simulink model "MSFartoystyring_path"  (R2018a)
settings: Solver=ode45  StartTime=tstart  StopTime=tstop  RelTol=1e-3  EnableMultiTasking=on
values from neighbouring files (symbols this model uses):
  c = 0    [run_heading.m]    (also in run_heading_controller.m = 1; run_heading_model.m; run_path.m = 1; run_path_crab.m)
  K_d = 2*zeta*w_n*(m + K_m) - d    [run_heading_controller.m]    (also in run_path.m)
  K_i = w_n / 10 * K_p    [run_heading_controller.m]    (also in run_path.m)
  K_p = (m+K_m)*w_n^2 - k    [run_heading_controller.m]    (also in run_path.m)
  n_max = (85*2*pi)/60    (= 8.90117918517)    [run_heading.m]    (also in run_heading_controller.m; run_heading_model.m; run_path.m; run_path_crab.m)
  p0 = zeros(2,1)    [run_heading.m]    (also in run_heading_controller.m; run_heading_model.m; run_path.m = [1000; 700]; run_path_crab.m = [1000; 700])
  psi0 = 0    [run_heading.m]    (also in run_heading_controller.m; run_heading_model.m; run_path.m = deg2rad(60); run_path_crab.m = deg2rad(-135))
  psi_d = deg2rad(10)    [run_path.m]    (also in run_path_crab.m; run_track.m)
  r0 = 0    [run_heading.m]    (also in run_heading_controller.m; run_heading_model.m; run_path.m; run_path_crab.m)
  tsamp = 10    [run_heading.m]    (also in run_heading_controller.m = 1; run_heading_model.m = 1; run_path.m; run_path_crab.m)
  v0 = [6.63 0]'    [run_heading.m]    (also in run_heading_controller.m; run_heading_model.m; run_path.m; run_path_crab.m)
undefined symbols (not defined in the file or in its folder): msfartoystyring, WP
libraries: simulink x2
settings Model: ExtModeAutoUpdateStatusClock=off  Creator=christh  LastModifiedBy=nicho
settings DataIOCC: LimitDataPoints=on  SaveFormat=Array  SignalLoggingSaveFormat=ModelDataLogs
settings OptimizationCC: ExpressionDepthLimit=2147483647  InitFltsAndDblsToZero=on  LifeSpan=inf
settings DebuggingCC: UnderspecifiedInitializationDetection=Classic  MergeDetectMultiDrivingBlocksExec=none  SolverPrmCheckMsg=warning  FcnCallInpInsideContextMsg=warning  StateNameClashWarn=warning  SFUnexpectedBacktrackingDiag=warning  SFNoUnconditionalDefaultTransitionDiag=warning  SFExecutionAtInitializationDiag=none
settings HardwareCC: ProdBitPerPointer=32  ProdBitPerSizeT=32  ProdBitPerPtrDiffT=32  ProdLargestAtomicFloat=None  ProdIntDivRoundTo=Undefined  ProdEndianess=Unspecified  ProdWordSize=32  ProdHWDeviceType=32-bit Generic
settings ModelReferenceCC: PropagateSignalLabelsOutOfModel=off
settings CodeAppCC: StateflowObjectComments=on
settings GRTTargetCC: TargetLangStandard=C89/C90 (ANSI)  GeneratePreprocessorConditionals=Disable all  CombineOutputUpdateFcns=off  GRTInterface=on
settings ConfigComp: CovMetricSettings=dw  CovHtmlReporting=on  CovSaveCumulativeToWorkspaceVar=on  CovSaveSingleToWorkspaceVar=on  CovExternalEMLEnable=off

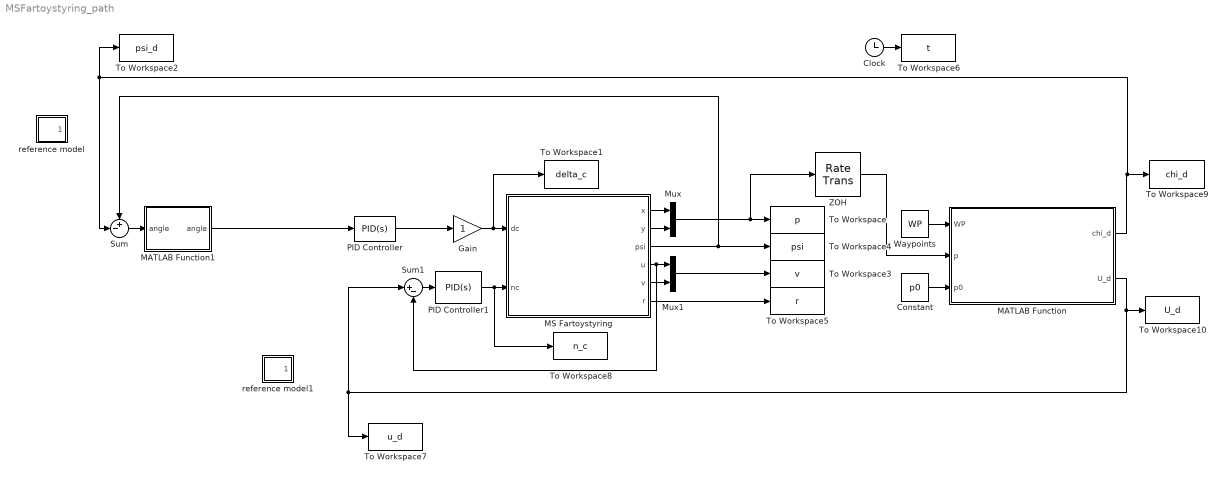
== system MSFartoystyring_path ==
  Clock : Clock
  Constant : Constant  Value=p0
  Gain : Gain
  MATLAB Function : MATLAB Function  TreatAsAtomicUnit=on
  MATLAB Function1 : MATLAB Function  TreatAsAtomicUnit=on
  MS Fartoystyring : Subsystem  mask(MS Fartoystyring for Assignment 3 G&C){x0=p0(1), y0=p0(2), u0=v0(1), v0=v0(2), psi0=psi0, r0=r0, c=c}
      mask prompts: x0 "x(t0) (m)"; y0 "y(t0) (m)"; u0 "u(t0) (m/s)"; v0 "v(t0) (m/s)"; psi0 "psi(t0) (rad)"; r0 "r(t0) (rad/s)"; c "current (0 or 1)"
      mask help:
      | Block corresponding to Figure 1 in the assignment text. Gives the response of the ship.
      |
      | The design speed of MS Fartoystyring is u=8.23 m/s.
      |
      | Input:
      | dc: commanded rudder (rad), dmax=25*pi/180
      | nc: commanded shaft speed (rad/s), nmax=85*2*pi/60
      |
      | Output:
      | x: north pos (m)
      | y: east pos (m)
      | u: surge (m/s)
      | v: sway (m/s)
      | psi: heading (rad)
      | r: yaw (rad/s)
      mask Help: Comments, bugs and help requests can be directed to the TA. Email on course website.
  Mux : Mux  Inputs=2
  Mux1 : Mux  Inputs=2
  PID Controller : simulink/Continuous/PID Controller  Controller=PID  TimeDomain=Continuous-time  SampleTime=-1  IntegratorMethod=Forward Euler  FilterMethod=Forward Euler  Form=Parallel  UseFilter=on  ControllerParametersSource=internal  P=K_p  I=K_i  D=K_d  N=0.0237516416222345  InitialConditionSource=internal  InitialConditionForIntegrator=0  InitialConditionForFilter=0  ExternalReset=none  LimitOutput=on  UpperSaturationLimit=inf  LowerSaturationLimit=-inf  LinearizeAsGain=on  AntiWindupMode=clamping  Kb=1  TrackingMode=off  Kt=1  PParamMin=[]  PParamMax=[]  IParamMin=[]  IParamMax=[]  DParamMin=[]  DParamMax=[]  NParamMin=[]  NParamMax=[]  KbParamMin=[]  KbParamMax=[]  KtParamMin=[]  KtParamMax=[]  POutMin=[]  POutMax=[]  IOutMin=[]  IOutMax=[]  DOutMin=[]  DOutMax=[]  NOutMin=[]  NOutMax=[]  KbOutMin=[]  KbOutMax=[]  KtOutMin=[]  KtOutMax=[]  IntegratorOutMin=[]  IntegratorOutMax=[]  FilterOutMin=[]  FilterOutMax=[]  SumOutMin=[]  SumOutMax=[]  SumI1OutMin=[]  SumI1OutMax=[]  SumI2OutMin=[]  SumI2OutMax=[]  SumI3OutMin=[]  SumI3OutMax=[]  SumDOutMin=[]  SumDOutMax=[]  SaturationOutMin=[]  SaturationOutMax=[]  IntegratorContinuousStateAttributes=''  IntegratorStateMustResolveToSignalObject=off  IntegratorRTWStateStorageClass=Auto  FilterContinuousStateAttributes=''  FilterStateMustResolveToSignalObject=off  FilterRTWStateStorageClass=Auto  DifferentiatorICPrevScaledInput=0  DifferentiatorOutMin=[]  DifferentiatorOutMax=[]  FilterDiffOutCoefMin=[]  FilterDiffOutCoefMax=[]  SumDenOutMin=[]  SumDenOutMax=[]  SumNumOutMin=[]  SumNumOutMax=[]  ReciprocalOutMin=[]  ReciprocalOutMax=[]  DivideOutMin=[]  DivideOutMax=[]  TunerSelectOption=Transfer Function Based (PID Tuner App)
  PID Controller1 : simulink/Continuous/PID Controller  Controller=PID  TimeDomain=Continuous-time  SampleTime=-1  IntegratorMethod=Forward Euler  FilterMethod=Forward Euler  Form=Parallel  UseFilter=on  ControllerParametersSource=internal  P=10  I=2  D=0  N=0.00193532941073824  InitialConditionSource=internal  InitialConditionForIntegrator=0  InitialConditionForFilter=0  ExternalReset=none  LimitOutput=on  UpperSaturationLimit=n_max  LowerSaturationLimit=-n_max  LinearizeAsGain=on  AntiWindupMode=clamping  Kb=1  TrackingMode=off  Kt=1  PParamMin=[]  PParamMax=[]  IParamMin=[]  IParamMax=[]  DParamMin=[]  DParamMax=[]  NParamMin=[]  NParamMax=[]  KbParamMin=[]  KbParamMax=[]  KtParamMin=[]  KtParamMax=[]  POutMin=[]  POutMax=[]  IOutMin=[]  IOutMax=[]  DOutMin=[]  DOutMax=[]  NOutMin=[]  NOutMax=[]  KbOutMin=[]  KbOutMax=[]  KtOutMin=[]  KtOutMax=[]  IntegratorOutMin=[]  IntegratorOutMax=[]  FilterOutMin=[]  FilterOutMax=[]  SumOutMin=[]  SumOutMax=[]  SumI1OutMin=[]  SumI1OutMax=[]  SumI2OutMin=[]  SumI2OutMax=[]  SumI3OutMin=[]  SumI3OutMax=[]  SumDOutMin=[]  SumDOutMax=[]  SaturationOutMin=[]  SaturationOutMax=[]  IntegratorContinuousStateAttributes=''  IntegratorStateMustResolveToSignalObject=off  IntegratorRTWStateStorageClass=Auto  FilterContinuousStateAttributes=''  FilterStateMustResolveToSignalObject=off  FilterRTWStateStorageClass=Auto  DifferentiatorICPrevScaledInput=0  DifferentiatorOutMin=[]  DifferentiatorOutMax=[]  FilterDiffOutCoefMin=[]  FilterDiffOutCoefMax=[]  SumDenOutMin=[]  SumDenOutMax=[]  SumNumOutMin=[]  SumNumOutMax=[]  ReciprocalOutMin=[]  ReciprocalOutMax=[]  DivideOutMin=[]  DivideOutMax=[]  TunerSelectOption=Transfer Function Based (PID Tuner App)
  Sum : Sum  Inputs=+-|
  Sum1 : Sum  Inputs=|+-
  To Workspace : ToWorkspace  VariableName=p  SampleTime=tsamp
  To Workspace1 : ToWorkspace  VariableName=delta_c  SampleTime=tsamp
  To Workspace10 : ToWorkspace  VariableName=U_d  SaveFormat=Timeseries  SampleTime=-1
  To Workspace2 : ToWorkspace  VariableName=psi_d  SampleTime=tsamp
  To Workspace3 : ToWorkspace  VariableName=v  SampleTime=tsamp
  To Workspace4 : ToWorkspace  VariableName=psi  SampleTime=tsamp
  To Workspace5 : ToWorkspace  VariableName=r  SampleTime=tsamp
  To Workspace6 : ToWorkspace  VariableName=t  SampleTime=tsamp
  To Workspace7 : ToWorkspace  VariableName=u_d  SampleTime=tsamp
  To Workspace8 : ToWorkspace  VariableName=n_c  SampleTime=tsamp
  To Workspace9 : ToWorkspace  VariableName=chi_d  SaveFormat=Timeseries  SampleTime=-1
  Waypoints : Constant  Value=WP
  ZOH : RateTransition  OutPortSampleTime=1
  reference model : Subsystem
  reference model1 : Subsystem
  wires:
  Clock/1 -> To Workspace6/1
  MS Fartoystyring/1(x) -> Mux/1
  MS Fartoystyring/2(y) -> Mux/2
  MS Fartoystyring/4(u) -> Sum1/2, Mux1/1
  MS Fartoystyring/5(v) -> Mux1/2
  Mux/1 -> ZOH/1, To Workspace/1
  MS Fartoystyring/6(r) -> To Workspace5/1
  Gain/1 -> MS Fartoystyring/1(dc), To Workspace1/1
  Sum/1 -> MATLAB Function1/1("angle ")
  MS Fartoystyring/3(psi) -> Sum/1, To Workspace4/1
  PID Controller1/1 -> To Workspace8/1, MS Fartoystyring/2(nc)
  Sum1/1 -> PID Controller1/1
  Mux1/1 -> To Workspace3/1
  MATLAB Function/2(U_d) -> To Workspace10/1, Sum1/1, To Workspace7/1
  Waypoints/1 -> MATLAB Function/1(WP)
  Constant/1 -> MATLAB Function/3(p0)
  ZOH/1 -> MATLAB Function/2(p)
  MATLAB Function/1(chi_d) -> Sum/2, To Workspace2/1, To Workspace9/1
  PID Controller/1 -> Gain/1
  MATLAB Function1/1(angle) -> PID Controller/1

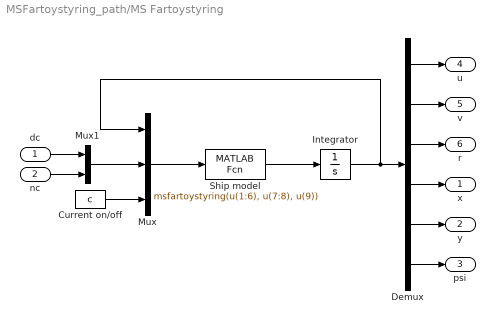
== system MSFartoystyring_path/MS Fartoystyring ==
  dc : Inport
  nc : Inport  Port=2
  Current on/off : Constant  Value=c
  Demux : Demux  Outputs=6
  Integrator : Integrator  InitialCondition=[u0 v0 r0 x0 y0 psi0]'
  Mux : Mux  Inputs=3
  Mux1 : Mux  Inputs=2
  Ship model : MATLABFcn  MATLABFcn=msfartoystyring(u(1:6), u(7:8), u(9))  OutputDimensions=6
  x : Outport
  y : Outport  Port=2
  psi : Outport  Port=3
  u : Outport  Port=4
  v : Outport  Port=5
  r : Outport  Port=6
  wires:
  Integrator/1 -> Mux/1, Demux/1
  Mux1/1 -> Mux/2
  dc/1 -> Mux1/1
  nc/1 -> Mux1/2
  Demux/1 -> u/1
  Demux/2 -> v/1
  Demux/3 -> r/1
  Demux/4 -> x/1
  Demux/5 -> y/1
  Demux/6 -> psi/1
  Current on/off/1 -> Mux/3
  Ship model/1 -> Integrator/1
  Mux/1 -> Ship model/1

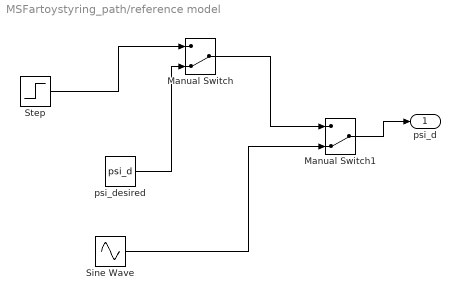
== system MSFartoystyring_path/reference model ==
  Manual Switch : ManualSwitch  CurrentSetting=0
  Manual Switch1 : ManualSwitch  CurrentSetting=0
  Sine Wave : Sin  Amplitude=0.4  Frequency=0.004  SampleTime=0
  Step : Step  Time=3000  After=15*pi/180  SampleTime=0
  psi_desired : Constant  Value=psi_d
  "psi_d " : Outport
  wires:
  psi_desired/1 -> Manual Switch/2
  Step/1 -> Manual Switch/1
  Sine Wave/1 -> Manual Switch1/2
  Manual Switch/1 -> Manual Switch1/1
  Manual Switch1/1 -> "psi_d "/1

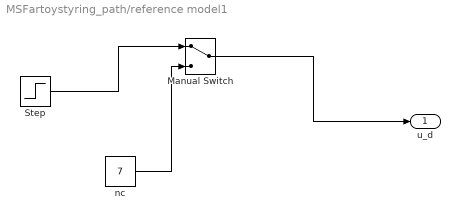
== system MSFartoystyring_path/reference model1 ==
  Manual Switch : ManualSwitch
  Step : Step  Time=1250  Before=3  After=7  SampleTime=0
  "nc " : Constant  Value=7
  "u_d " : Outport
  wires:
  "nc "/1 -> Manual Switch/2
  Step/1 -> Manual Switch/1
  Manual Switch/1 -> "u_d "/1

== matlab function MSFartoystyring_path/MATLAB Function1 ==
  data: angle input; angle output
function angle = ssa(angle)
    angle = mod(angle + pi, 2*pi) - pi;

== matlab function MSFartoystyring_path/MATLAB Function ==
  settings: updateMethod=DISCRETE
  data: WP input; chi_d output; p input; U_d output; p0 input
function [chi_d, U_d] = fcn(WP, p, p0)
    [chi_d, U_d] = los(WP, p, p0);
end
